simulink model "Universal_continuous_simulation_75"  (Simulink 7.0)
settings: Solver=ode45  StartTime=0.0  StopTime=simulation_horizon  RelTol=1e-6  AbsTol=1e-6
values from neighbouring files (symbols this model uses):
  A = Phi    [MMCE.m]
  B = Gamma    [MMCE.m]
  Cm = Cmm    [MMCE.m]
  F = zeros(n)    [MMCE.m]    (also in yalmip_lmi_reg.m = F + set(kron(Lreg,Y) + kron(Mreg,(A*Y-B*W)') + kron(Mreg',(A)
  G = zeros(n,q)    [MMCE.m]
  H = zeros(n)    [MMCE.m]
  J = zeros(n,p)    [MMCE.m]
  K = zeros(n,q)    [MMCE.m]
  L1 = L    [MMCE.m]
  L2 = zeros(p,q)    [MMCE.m]
  M = [A-lambdades(i)*eye(n) -B]    [Choice_Eigenvec_Paramvec.m]    (also in Falb_Wolovich_or_Roppenecker.m = inv(Dstar)*diag([knum]); MMCE.m = inv(G_CL),)
  n = size(A,1)    [Becker_Ostertag.m]    (also in Falb_Wolovich_or_Roppenecker.m; MMCE.m; Responses.m = size(A_CL,1); Roppenecker.m)
  p = size(B,2)    [Becker_Ostertag.m]    (also in Falb_Wolovich_or_Roppenecker.m; MMCE.m = size(Bc,2); Responses.m; Roppenecker.m)
  p_load = 1    [MMCE.m]
  p_measurements = -0.5    [MMCE.m]
  re = size(Em,2)    [MMCE.m]
  Sc = zeros(qc, q)    [MMCE.m]
  Si = zeros(q,q)    [MMCE.m]
  simulation_horizon = 15*Ts    (= 15)    [MMCE.m]
  start_p_load = 5*Ts    (= 5)    [MMCE.m]
  start_p_measurements = 10*Ts    (= 10)    [MMCE.m]
  start_reference = 0    [MMCE.m]
  x0 = xx0    [MMCE.m]    (also in Responses.m = as above) (Y/N)? [N] --> ','s'); yalmip_lmi_reg.m = input('  Enter a real number:  '))
  yr = 1    [MMCE.m]
  z0 = 0    [MMCE.m]
libraries: simulink x5
settings Model: Creator=Eric  LastModifiedBy=Eric  ExtModeTrigMode=oneshot  ExtModeArmWhenConnect=off
settings SolverCC: InitialStep=0.001
settings DataIOCC: LimitDataPoints=off  SignalLoggingName=sigsOut
settings OptimizationCC: BooleanDataType=off
settings DebuggingCC: SaveWithParameterizedLinksMsg=none  SignalResolutionControl=TryResolveAllWithWarning  SolverPrmCheckMsg=none  MultiTaskDSMMsg=warning  MultiTaskCondExecSysMsg=none  StrictBusMsg=None
settings HardwareCC: TargetUnknown=on
settings RTWCC: IncludeERTFirstTime=on
settings GRTTargetCC: TargetFcnLib=ansi_tfl_tmw.mat

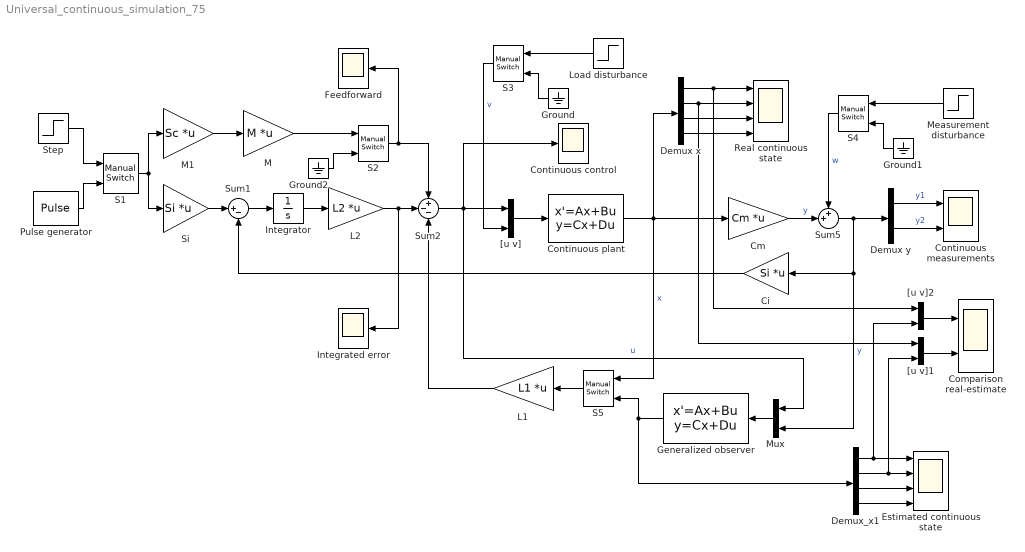
== system Universal_continuous_simulation_75 ==
  Ci : Gain  Orientation=left  Gain=Si  Multiplication=Matrix(K*u)  ParameterDataType=sfix(16)  ParameterScaling=2^0  OutDataType=sfix(16)  OutScaling=2^0  SaturateOnIntegerOverflow=on
  Cm : Gain  Gain=Cm  Multiplication=Matrix(K*u)  ParameterDataType=sfix(16)  ParameterScaling=2^0  OutDataType=sfix(16)  OutScaling=2^0  SaturateOnIntegerOverflow=on
  Comparison real-estimate : Scope  NumInputPorts=2
      settings: YMin=-0.1~-0.2  YMax=0.3~0.2  SaveName=CompareScope  MaxDataPoints=100000
  Continuous measurements : Scope  NumInputPorts=2
      settings: YMin=-0.5~-0.15  YMax=2~0.05  SaveName=MeasurementScope  MaxDataPoints=100000
  Continuous control : Scope
      settings: YMin=-0.5  YMax=0.5  SaveName=ControlScope  MaxDataPoints=100000
  Continuous plant : StateSpace  A=A  B=[B E]  C=eye(n)  D=zeros(n,p+re)  X0=[x0]
  Demux x : Demux  Outputs=n
  Demux y : Demux  Outputs=q
  Demux_x1 : Demux  Outputs=n
  Estimated continuous state : Scope  NumInputPorts=4
      settings: YMin=-0.1~-0.2~-0.15~-5  YMax=0.3~0.2~0.05~5  SaveName=EstimateScope  MaxDataPoints=100000
  Feedforward : Scope
      settings: YMin=-2  YMax=4  SaveName=ScopeData3  MaxDataPoints=100000
  Generalized observer : StateSpace  Orientation=left  A=F  B="[J  G]"  C=H  D="[zeros(n,p)  K]"  X0=[z0]
  Ground : Ground  Orientation=left
  Ground1 : Ground  Orientation=left
  Ground2 : Ground
  Integrated error : Scope
      settings: YMin=-2  YMax=0  MaxDataPoints=100000
  Integrator : Integrator  InitialCondition=[0]
  L1 : Gain  Orientation=left  Gain=L1  Multiplication=Matrix(K*u)  ParameterDataType=sfix(16)  ParameterScaling=2^0  OutDataType=sfix(16)  OutScaling=2^0  SaturateOnIntegerOverflow=on
  L2 : Gain  Gain=L2  Multiplication=Matrix(K*u)  ParameterDataType=sfix(16)  ParameterScaling=2^0  OutDataType=sfix(16)  OutScaling=2^0  SaturateOnIntegerOverflow=on
  Load disturbance : Step  Orientation=left  Time=start_p_load  Before=[0]  After=p_load  SampleTime=0
  M : Gain  Gain=M  Multiplication=Matrix(K*u)  ParameterDataType=sfix(16)  ParameterScaling=2^0  OutDataType=sfix(16)  OutScaling=2^0  SaturateOnIntegerOverflow=on
  M1 : Gain  Gain=Sc  Multiplication=Matrix(K*u)  ParameterDataType=sfix(16)  ParameterScaling=2^0  OutDataType=sfix(16)  OutScaling=2^0  SaturateOnIntegerOverflow=on
  Measurement disturbance : Step  Orientation=left  Time=start_p_measurements  Before=[0]  After=p_measurements  SampleTime=0
  Mux : Mux  Orientation=left  Inputs=2
  Pulse generator : DiscretePulseGenerator  PulseType=Time based  Amplitude=yr  Period=simulation_horizon/2.5  PulseWidth=50
  Real continuous state : Scope  NumInputPorts=4
      settings: YMin=-0.1~-0.2~-0.15~-5  YMax=0.3~0.2~0.05~5  SaveName=StateScope  MaxDataPoints=100000
  S1 : simulink/Signal Routing/Manual Switch  SystemSampleTime=-1  sw=1  action=0  varsize=off
  S2 : simulink/Signal Routing/Manual Switch  SystemSampleTime=-1  sw=1  action=0  varsize=off
  S3 : simulink/Signal Routing/Manual Switch  Orientation=left  SystemSampleTime=-1  sw=0  action=0  varsize=off
  S4 : simulink/Signal Routing/Manual Switch  Orientation=left  SystemSampleTime=-1  sw=0  action=0  varsize=off
  S5 : simulink/Signal Routing/Manual Switch  Orientation=left  SystemSampleTime=-1  sw=1  action=0  varsize=off
  Si : Gain  Gain=Si  Multiplication=Matrix(K*u)  ParameterDataType=sfix(16)  ParameterScaling=2^0  OutDataType=sfix(16)  OutScaling=2^0  SaturateOnIntegerOverflow=on
  Step : Step  Time=start_reference  Before=[0]  After=yr  SampleTime=0
  Sum1 : Sum  Inputs=|+-  OutDataType=sfix(16)  OutScaling=2^0  SaturateOnIntegerOverflow=on  InputSameDT=on
  Sum2 : Sum  Inputs=+--  OutDataType=sfix(16)  OutScaling=2^0  SaturateOnIntegerOverflow=on  InputSameDT=on
  Sum5 : Sum  Inputs=++|  OutDataType=sfix(16)  OutScaling=2^0  SaturateOnIntegerOverflow=on
  "[u v]" : Mux  Inputs=2
  "[u v]1" : Mux  Inputs=2
  "[u v]2" : Mux  Inputs=2
  wires:
  Sum1/1 -> Integrator/1
  Integrator/1 -> L2/1
  Demux x/2 -> Real continuous state/2, "[u v]1"/1
  Demux x/1 -> Real continuous state/1, "[u v]2"/1
  Load disturbance/1 -> S3/1
  S3/1 -> "[u v]"/2  "v"
  Ground/1 -> S3/2
  Continuous plant/1 -> Cm/1, Demux x/1, S5/1  "x"
  Ground1/1 -> S4/2
  Sum2/1 -> "[u v]"/1, Continuous control/1, Mux/1  "u"
  "[u v]"/1 -> Continuous plant/1
  L1/1 -> Sum2/3
  S2/1 -> Sum2/1, Feedforward/1
  Ground2/1 -> S2/2
  M/1 -> S2/1
  Measurement disturbance/1 -> S4/1
  L2/1 -> Sum2/2, Integrated error/1
  Ci/1 -> Sum1/2
  S5/1 -> L1/1
  Mux/1 -> Generalized observer/1
  Generalized observer/1 -> Demux_x1/1, S5/2
  Demux_x1/1 -> Estimated continuous state/1, "[u v]2"/2
  Demux_x1/2 -> Estimated continuous state/2, "[u v]1"/2
  Step/1 -> S1/1
  Pulse generator/1 -> S1/2
  Demux y/1 -> Continuous measurements/1  "y1"
  "[u v]2"/1 -> Comparison real-estimate/1
  "[u v]1"/1 -> Comparison real-estimate/2
  S4/1 -> Sum5/1  "w"
  Cm/1 -> Sum5/2  "y"
  Sum5/1 -> Demux y/1, Mux/2, Ci/1  "y"
  Demux y/2 -> Continuous measurements/2  "y2"
  Demux_x1/4 -> Estimated continuous state/4
  Si/1 -> Sum1/1
  S1/1 -> Si/1, M1/1
  M1/1 -> M/1
  Demux x/3 -> Real continuous state/3
  Demux x/4 -> Real continuous state/4
  Demux_x1/3 -> Estimated continuous state/3
